simulink model "D1_LookUp"  (R2024b)
settings: Solver=VariableStepAuto  StartTime=0.0  StopTime=10.0  RelTol=1e-3
settings Model: Creator=Ahmad  LastModifiedBy=Ahmad

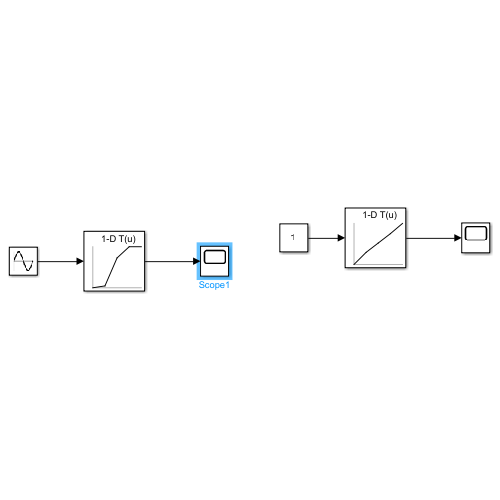
[thumbnail: Simulink's stored preview of the top-level diagram]
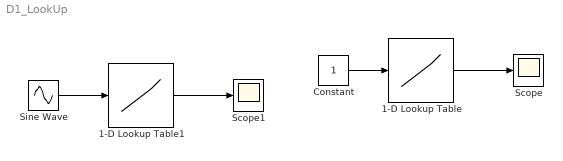
== system D1_LookUp ==
  1-D Lookup Table : Lookup_n-D  NumberOfTableDimensions=1  BreakpointsForDimension1=[0,20,40,60,80]  Table=[1,2.5,3.7,4.9,6.2]  InternalRulePriority=Speed  RndMeth=Simplest
  1-D Lookup Table1 : Lookup_n-D  NumberOfTableDimensions=1  BreakpointsForDimension1=[0,20,40,60,80]  Table=[0.5,0.75,3.7,4.9,4.9]  InternalRulePriority=Speed  RndMeth=Simplest
  Constant : Constant
  Scope : Scope
  Scope1 : Scope
  Sine Wave : Sin  SampleTime=0
  wires:
  Constant/1 -> 1-D Lookup Table/1
  1-D Lookup Table/1 -> Scope/1
  1-D Lookup Table1/1 -> Scope1/1
  Sine Wave/1 -> 1-D Lookup Table1/1
